simulink model "Aufgabe7_Bausteine"  (R2016a)
settings: Solver=ode45  StartTime=0.0  StopTime=10.0  RelTol=1e-3
libraries: dspstat3 x2, commdigbbndam3 x1, simulink_extras x1, commsink2 x1
settings Model: Creator=Bornitz  LastModifiedBy=Bornitz
settings DataIOCC: LimitDataPoints=on  SaveFormat=Array
settings OptimizationCC: ExpressionDepthLimit=2147483647
settings DebuggingCC: UnderspecifiedInitializationDetection=Classic  MergeDetectMultiDrivingBlocksExec=none  SolverPrmCheckMsg=warning  AllowSymbolicDim=off  StateNameClashWarn=warning  StrictBusMsg=Warning
settings HardwareCC: ProdBitPerPointer=32  ProdLargestAtomicFloat=None  ProdIntDivRoundTo=Undefined  ProdEndianess=Unspecified  ProdWordSize=32  ProdHWDeviceType=32-bit Generic
settings ModelReferenceCC: PropagateSignalLabelsOutOfModel=off
settings SFSimCC: SimParseCustomCode=off
settings GRTTargetCC: CombineOutputUpdateFcns=off  GRTInterface=on
settings ConfigComp: CovModelRefEnable=Off

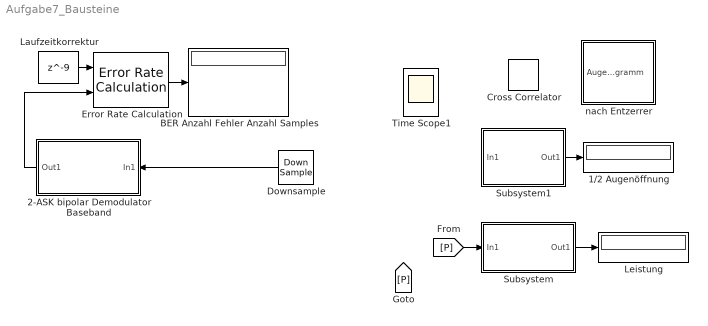
== system Aufgabe7_Bausteine ==
  1/2 Augenöffnung : Display
  2-ASK bipolar Demodulator Baseband : Subsystem
      mask Display:
      | plot(0,0,100,100,[20+1.5*[[0:.8:10] [10:1.6:20] [20:.8:30]] 65 65 65 65+10*[0 1 1 2 2 3]],[85+10*[sin([0:.8:10]*pi*2/5) sin([10:1.6:20]*pi/5) sin([20:.8:30]*pi*2/5)] 85 99 75 85+8*[1 1 -1 -1 1 1]]);
      | disp('\nGeneral\nASK-Demodulator')
  BER Anzahl Fehler Anzahl Samples : Display
      settings: Format=short_e  Decimation=2
  Cross Correlator : simulink_extras/Additional Sinks/Cross Correlator  npts=100  HowOften=50  sampleT=0.0002
  Downsample : DownSample  N=16  RateOptions=Allow multirate processing
  Error Rate Calculation : commsink2/Error Rate Calculation  N=0  st_delay=100  cp_mode=Entire frame  subframe=1  PMode=Port  WsName=ErrorVec  RsMode2=off  stop=off  numErr=100  maxBits=1e6
  Laufzeitkorrektur : Delay  DelayLength=9  InitialCondition=0  InputProcessing=Columns as channels (frame based)
  "Leistung " : Display
  Subsystem : Subsystem
      mask Display: disp('Leistungsmessung ')
  Subsystem1 : Subsystem
      mask Display:
      | image('eye.bmp','center')
      | disp('\n\n\nAugenöffnung')
  Time Scope1 : Scope
  nach Entzerrer : Subsystem
  wires:
  Error Rate Calculation/1 -> BER Anzahl Fehler Anzahl Samples/1
  Laufzeitkorrektur/1 -> Error Rate Calculation/1
  Downsample/1 -> 2-ASK bipolar Demodulator Baseband/1(In1)
  2-ASK bipolar Demodulator Baseband/1(Out1) -> Error Rate Calculation/2
  [P] -> Subsystem/1(In1)
  Subsystem/1(Out1) -> "Leistung "/1
  Subsystem1/1(Out1) -> 1/2 Augenöffnung/1

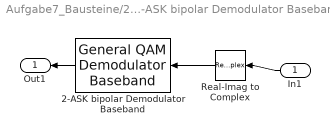
== system Aufgabe7_Bausteine/2-ASK bipolar Demodulator Baseband ==
  In1 : Inport
  2-ASK bipolar Demodulator Baseband : commdigbbndam3/General QAM Demodulator Baseband  SigCon=sigdem2  OutType=Integer  DecType=Hard decision  VarSource=Dialog  Variance=1  outDtypeBit=Inherit via internal rule  outDtype=Inherit via internal rule  roundingMode=Floor  overflowMode=Wrap  OvFlMode=off  OvFlModeLastStrValue=off  sigConstWordLen=16  sigConstDataTypeStr=Inherit: Same word length as input  sigConstLastDataTypeStr=Inherit: Same word length as input  accum1WordLen=32  accum1FracLen=30  prodInWordLen=32  prodInFracLen=30  prodInDataTypeStr=Inherit: Same as accumulator 1  prodInLastDataTypeStr=Inherit: Same as accumulator 1  prodOutWordLen=32  prodOutFracLen=30  accum2WordLen=32  accum2FracLen=30  accum3WordLen=32  accum3FracLen=30  nsiWordLen=32  nsiFracLen=30  nsiDataTypeStr=Inherit: Same as accumulator 3  nsiLastDataTypeStr=Inherit: Same as accumulator 3  invn0WordLen=16  invn0FracLen=8  invn0DataTypeStr=Inherit: Same word length as input  invn0LastDataTypeStr=Inherit: Same word length as input  outputWordLen=32  outputFracLen=30
  Real-Imag to Complex : RealImagToComplex  Input=Real
  Out1 : Outport
  wires:
  Real-Imag to Complex/1 -> 2-ASK bipolar Demodulator Baseband/1
  In1/1 -> Real-Imag to Complex/1
  2-ASK bipolar Demodulator Baseband/1 -> Out1/1

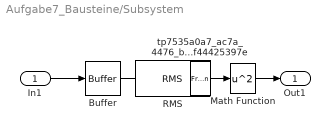
== system Aufgabe7_Bausteine/Subsystem ==
  In1 : Inport
  Buffer : Buffer  N=4000  TreatMby1Signals=One channel  OutputFrames=off
  Math Function : Math  Operator=square  SaturateOnIntegerOverflow=on
  RMS : dspstat3/RMS  run=off  reset_popup=None  InputProcessing=Columns as channels (frame based)  directionMode=Entire input  dimension=1
  tp7535a0a7_ac7a_4476_be6b_98f44425397e : FrameConversion  InheritSamplingMode=off
  Out1 : Outport
  wires:
  tp7535a0a7_ac7a_4476_be6b_98f44425397e/1 -> RMS/1
  Buffer/1 -> tp7535a0a7_ac7a_4476_be6b_98f44425397e/1
  Math Function/1 -> Out1/1
  In1/1 -> Buffer/1
  RMS/1 -> Math Function/1

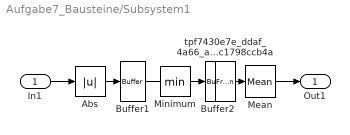
== system Aufgabe7_Bausteine/Subsystem1 ==
  In1 : Inport
  Abs : Abs
  Buffer1 : Buffer  N=20  V=4  TreatMby1Signals=One channel  OutputFrames=off
  Buffer2 : Buffer  N=20  V=4  TreatMby1Signals=One channel
  Mean : dspstat3/Mean  run=off  reset_popup=None  InputProcessing=Columns as channels (frame based)  directionMode=Each column  dimension=1  roiEnable=off  roiType=Rectangles  roiPortion=Entire ROI  roiOutput=Individual statistics for each ROI  roiFlag=off  outputDataTypeStr=Inherit: Same as accumulator  outputLastDataTypeStr=Inherit: Same as accumulator  outputMin=[]  outputMax=[]  roundingMode=Floor  overflowMode=off
  Minimum : MinMax
  tpf7430e7e_ddaf_4a66_a69d_5cc1798ccb4a : FrameConversion  InheritSamplingMode=off
  Out1 : Outport
  wires:
  tpf7430e7e_ddaf_4a66_a69d_5cc1798ccb4a/1 -> Minimum/1
  Buffer1/1 -> tpf7430e7e_ddaf_4a66_a69d_5cc1798ccb4a/1
  Mean/1 -> Out1/1
  In1/1 -> Abs/1
  Buffer2/1 -> Mean/1
  Minimum/1 -> Buffer2/1
  Abs/1 -> Buffer1/1

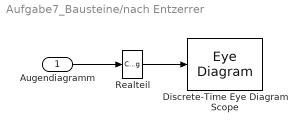
== system Aufgabe7_Bausteine/nach Entzerrer ==
  Augendiagramm : Inport
  Discrete-Time Eye Diagram Scope : EyeDiagram  Tag=EyeDiagram
  Realteil : ComplexToRealImag  Output=Real
  wires:
  Realteil/1 -> Discrete-Time Eye Diagram Scope/1
  Augendiagramm/1 -> Realteil/1
